simulink model "P5"  (R2019a)
settings: Solver=VariableStepAuto  StartTime=0.0  StopTime=10.0  RelTol=1e-3
settings Model: Creator=ADMIN  LastModifiedBy=ADMIN

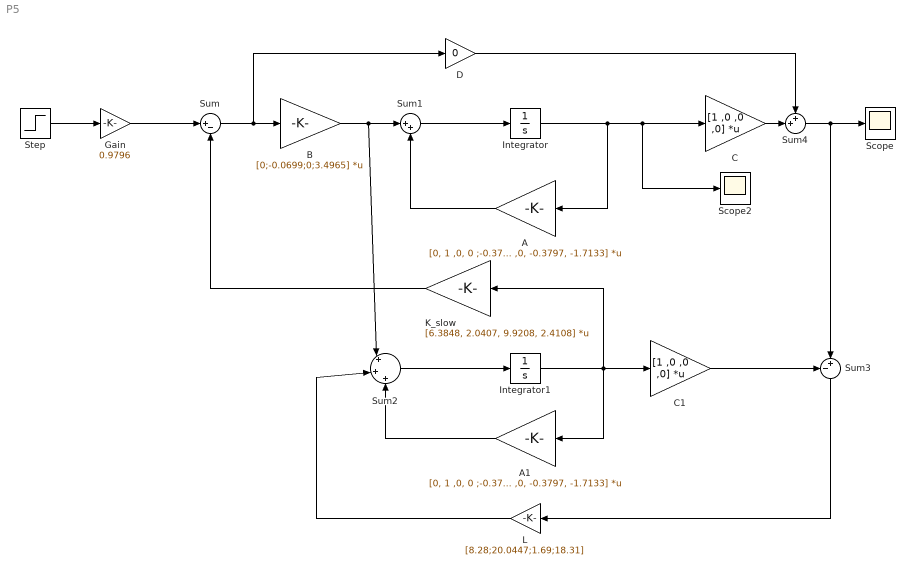
== system P5 ==
  A : Gain  Gain=[0, 1 ,0, 0 ;-0.378 ,0 ,7.0147 ,0.0343;0, 0, 0, 1; 18.9001 ,0, -0.3797, -1.7133]  Multiplication=Matrix(K*u) (u vector)
  A1 : Gain  Gain=[0, 1 ,0, 0 ;-0.378 ,0 ,7.0147 ,0.0343;0, 0, 0, 1; 18.9001 ,0, -0.3797, -1.7133]  Multiplication=Matrix(K*u) (u vector)
  B : Gain  Gain=[0;-0.0699;0;3.4965]  Multiplication=Matrix(K*u) (u vector)
  C : Gain  Gain=[1 ,0 ,0 ,0]  Multiplication=Matrix(K*u) (u vector)
  C1 : Gain  Gain=[1 ,0 ,0 ,0]  Multiplication=Matrix(K*u) (u vector)
  D : Gain  Gain=0
  Gain : Gain  Gain=0.9796
  Integrator : Integrator
  Integrator1 : Integrator
  K_slow : Gain  Gain=[6.3848, 2.0407, 9.9208, 2.4108]  Multiplication=Matrix(K*u) (u vector)
  L : Gain  Gain=[8.28;20.0447;1.69;18.31]
  Scope : Scope
  Scope2 : Scope
  Step : Step  Time=0  After=0.1  SampleTime=0
  Sum : Sum  Inputs=|+-
  Sum1 : Sum  Inputs=|++
  Sum2 : Sum  Inputs=|+|+|+
  Sum3 : Sum  Inputs=-+|
  Sum4 : Sum  Inputs=++|
  wires:
  Sum/1 -> B/1, D/1
  K_slow/1 -> Sum/2
  Gain/1 -> Sum/1
  Step/1 -> Gain/1
  Sum4/1 -> Scope/1, Sum3/2
  C/1 -> Sum4/2
  Integrator/1 -> A/1, C/1, Scope2/1
  A/1 -> Sum1/2
  D/1 -> Sum4/1
  Sum1/1 -> Integrator/1
  B/1 -> Sum2/1, Sum1/1
  Sum2/1 -> Integrator1/1
  Integrator1/1 -> K_slow/1, C1/1, A1/1
  C1/1 -> Sum3/1
  Sum3/1 -> L/1
  A1/1 -> Sum2/3
  L/1 -> Sum2/2
